simulink model "PCMbackup"  (R2018b)
settings: Solver=VariableStepAuto  StartTime=0.0  StopTime=160  RelTol=1e-3
libraries: commsrccod2 x3, commutil2 x3, dsparch4 x2, commsink2 x1, commchan3 x1
settings Model: Creator=lance  LastModifiedBy=lance

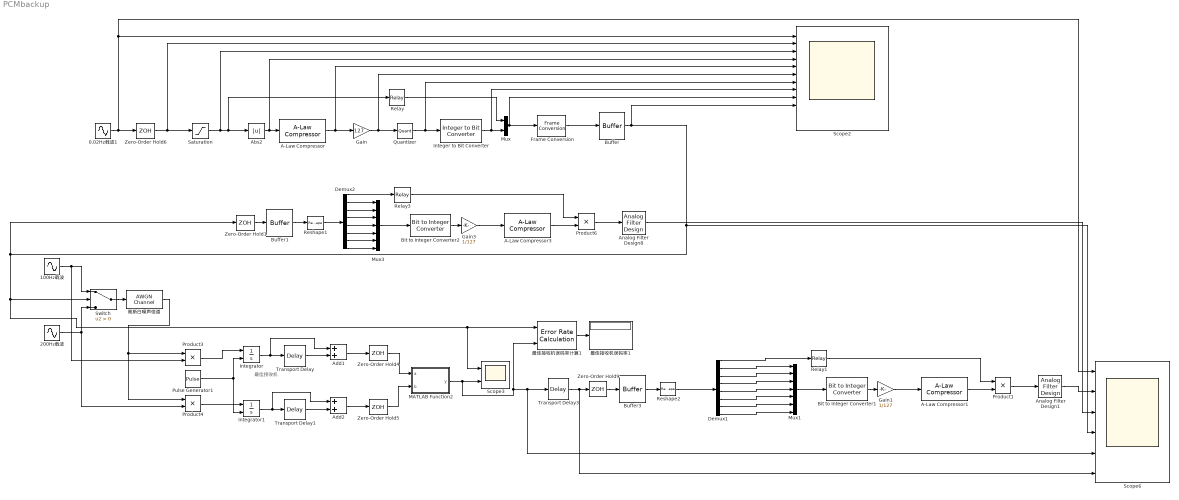
== system PCMbackup ==
  note: 最佳接收机
  0.02Hz载波1 : Sin  Frequency=0.05*2*pi  SampleTime=0.0001
  100Hz载波 : Sin  Frequency=100*2*pi  SampleTime=0.0001
  200Hz载波 : Sin  Frequency=200*2*pi  SampleTime=0.0001
  A-Law Compressor : commsrccod2/A-Law Compressor  A=87.6  V=1
      settings: SourceProductName=Communications System Toolbox  SourceProductBaseCode=CM
  A-Law Compressor1 : commsrccod2/A-Law Compressor  A=87.6  V=1
      settings: SourceProductName=Communications System Toolbox  SourceProductBaseCode=CM
  A-Law Compressor3 : commsrccod2/A-Law Compressor  A=87.6  V=1
      settings: SourceProductName=Communications System Toolbox  SourceProductBaseCode=CM
  Abs2 : Abs
  Add1 : Sum
  Add2 : Sum
  Analog Filter Design1 : dsparch4/Analog Filter Design  method=Butterworth  filttype=Lowpass  N=8  Wlo=0.1*2*pi  Whi=210*2*pi  Rp=2  Rs=40
  Analog Filter Design8 : dsparch4/Analog Filter Design  method=Butterworth  filttype=Lowpass  N=8  Wlo=0.1*pi  Whi=210*2*pi  Rp=2  Rs=40
  Bit to Integer Converter1 : commutil2/Bit to Integer Converter  nbits=7  bitOrder=MSB first  signedOutputValues=Unsigned  outDtype=Inherit via internal rule  outDtypeSigned=Inherit via internal rule
  Bit to Integer Converter2 : commutil2/Bit to Integer Converter  nbits=7  bitOrder=MSB first  signedOutputValues=Unsigned  outDtype=Inherit via internal rule  outDtypeSigned=Inherit via internal rule
  Buffer : Buffer  N=1  OutputFrames=off
  Buffer1 : Buffer  N=8  OutputFrames=off
  Buffer3 : Buffer  N=8  OutputFrames=off
  Demux1 : Demux  Outputs=8
  Demux2 : Demux  Outputs=8
  Frame Conversion : FrameConversion
  Gain : Gain  Gain=127
  Gain1 : Gain  Gain=1/127  SampleTime=0.2
  Gain3 : Gain  Gain=1/127  SampleTime=0.2
  Integer to Bit Converter : commutil2/Integer to Bit Converter  nbits=7  signedInputValues=Unsigned  bitOrder=MSB first  outDtype=Inherit via internal rule
  Integrator : Integrator  ExternalReset=rising
  Integrator1 : Integrator  ExternalReset=rising
  MATLAB Function2 : MATLAB Function  TreatAsAtomicUnit=on
  Mux : Mux  Inputs=2
  Mux1 : Mux  Inputs=7
  Mux3 : Mux  Inputs=7
  Product1 : Product  SampleTime=0.001  RndMeth=Zero
  Product3 : Product
  Product4 : Product
  Product6 : Product  SampleTime=0.001  RndMeth=Zero
  Pulse Generator1 : DiscretePulseGenerator  PulseType=Time based  Period=0.2
  Quantizer : Quantizer  QuantizationInterval=1
  Relay : Relay
  Relay1 : Relay  OffOutputValue=-1  SampleTime=0.001
  Relay3 : Relay  OffOutputValue=-1  SampleTime=0.001
  Reshape1 : Reshape
  Reshape2 : Reshape
  Saturation : Saturate  UpperLimit=1  LowerLimit=-1
  Scope2 : Scope  NumInputPorts=12
  Scope3 : Scope  NumInputPorts=2
  Scope6 : Scope  NumInputPorts=6
  Switch : Switch  Criteria=u2 > Threshold
  Transport Delay : TransportDelay  DelayTime=0.02
  Transport Delay1 : TransportDelay  DelayTime=0.02
  Transport Delay3 : TransportDelay  DelayTime=1.4
  Zero-Order Hold{1,4..5,9} (4 alike) : ZeroOrderHold  SampleTime=0.2
  Zero-Order Hold6 : ZeroOrderHold  SampleTime=1.6
  最佳接收机误码率1 : Display
  最佳接收机误码率计算1 : commsink2/Error Rate Calculation  N=1  st_delay=0  cp_mode=Entire frame  subframe=[]  PMode=Port  WsName=ErrorVec  RsMode2=off  stop=off  numErr=100  maxBits=1e6
  "高斯白噪声信道 " : commchan3/AWGN Channel  InputProcessing=Columns as channels (frame based)  seed=67  noiseMode="Signal to noise ratio  (SNR)"  EbNodB=1  EsNodB=10  SNRdB=-18  bitsPerSym=1  Ps=1  Tsym=1  variance=1
  wires:
  Gain/1 -> Scope2/6, Quantizer/1
  Integer to Bit Converter/1 -> Scope2/8, Mux/2
  A-Law Compressor/1 -> Scope2/5, Gain/1
  Relay/1 -> Mux/1
  Quantizer/1 -> Scope2/7, Integer to Bit Converter/1
  Saturation/1 -> Scope2/3, Relay/1, Abs2/1
  0.02Hz载波1/1 -> Scope6/1, Scope2/1, Zero-Order Hold6/1
  Abs2/1 -> Scope2/4, A-Law Compressor/1
  Zero-Order Hold6/1 -> Scope2/2, Saturation/1
  Mux3/1 -> Bit to Integer Converter2/1
  Demux2/1 -> Relay3/1
  Gain3/1 -> A-Law Compressor3/1
  Relay3/1 -> Product6/1
  Demux2/4 -> Mux3/3
  Bit to Integer Converter2/1 -> Gain3/1
  Demux2/5 -> Mux3/4
  Demux2/7 -> Mux3/6
  Demux2/2 -> Mux3/1
  Demux2/6 -> Mux3/5
  Demux2/3 -> Mux3/2
  A-Law Compressor3/1 -> Product6/2
  Mux/1 -> Frame Conversion/1, Scope2/9
  Demux2/8 -> Mux3/7
  Product6/1 -> Analog Filter Design8/1
  Frame Conversion/1 -> Buffer/1
  Zero-Order Hold1/1 -> Buffer1/1
  Buffer1/1 -> Reshape1/1
  Reshape1/1 -> Demux2/1
  Demux1/4 -> Mux1/3
  最佳接收机误码率计算1/1 -> 最佳接收机误码率1/1
  Switch/1 -> "高斯白噪声信道 "/1
  Gain1/1 -> A-Law Compressor1/1
  Integrator1/1 -> Add2/1, Transport Delay1/1
  Product4/1 -> Integrator1/1
  "高斯白噪声信道 "/1 -> Product4/1, Product3/1
  Integrator/1 -> Add1/1, Transport Delay/1
  Pulse Generator1/1 -> Integrator1/2, Integrator/2
  100Hz载波/1 -> Product3/2, Switch/1
  200Hz载波/1 -> Switch/3, Product4/2
  Add2/1 -> Zero-Order Hold5/1
  Relay1/1 -> Product1/1
  Zero-Order Hold5/1 -> MATLAB Function2/2(b)
  Demux1/6 -> Mux1/5
  A-Law Compressor1/1 -> Product1/2
  Product3/1 -> Integrator/1
  Demux1/8 -> Mux1/7
  Demux1/1 -> Relay1/1
  Buffer3/1 -> Reshape2/1
  Zero-Order Hold9/1 -> Buffer3/1
  Product1/1 -> Analog Filter Design1/1
  Add1/1 -> Zero-Order Hold4/1
  Reshape2/1 -> Demux1/1
  Demux1/3 -> Mux1/2
  Buffer/1 -> Zero-Order Hold1/1, Switch/2, Scope3/1, 最佳接收机误码率计算1/1, Scope6/4, Scope2/10
  Demux1/5 -> Mux1/4
  Transport Delay/1 -> Add1/2
  Demux1/7 -> Mux1/6
  Demux1/2 -> Mux1/1
  MATLAB Function2/1(y) -> Scope6/5, Transport Delay3/1, 最佳接收机误码率计算1/2, Scope3/2
  Transport Delay1/1 -> Add2/2
  Bit to Integer Converter1/1 -> Gain1/1
  Zero-Order Hold4/1 -> MATLAB Function2/1(a)
  Mux1/1 -> Bit to Integer Converter1/1
  Transport Delay3/1 -> Scope6/6, Zero-Order Hold9/1
  Analog Filter Design1/1 -> Scope6/2
  Analog Filter Design8/1 -> Scope6/3

== matlab function PCMbackup/MATLAB Function2 ==
  data: a input; y output; b input
function y = fcn(a, b)
if(a>b)
    y=1;
else
    y=0;
end
